simulink model "ResolvedMotion_Example"  (R2015b)
settings: Solver=ode45  StartTime=0.0  StopTime=10.0  MaxStep=1e-2  RelTol=1e-9  AbsTol=1e-9
InitFcn:
  | ResolvedMotion_Example_Init
values from neighbouring files (symbols this model uses):
  M0 = H0*q0dot0+H0m*qmdot0    [ResolvedMotion_Example_Init.m]
  qmdot0 = zeros(4,1)    [ResolvedMotion_Example_Init.m]
libraries: SPART_Lib x3, aerolibtransform2 x2, simulink x1
settings Model: Creator=Josep  LastModifiedBy=Josep
settings DataIOCC: SaveFormat=Array
settings HardwareCC: ProdBitPerPointer=32  ProdLargestAtomicFloat=None  ProdIntDivRoundTo=Undefined  ProdEndianess=Unspecified  ProdWordSize=32  ProdHWDeviceType=32-bit Generic
settings GRTTargetCC: GeneratePreprocessorConditionals=Disable all
settings ConfigComp: CovModelRefEnable=Off

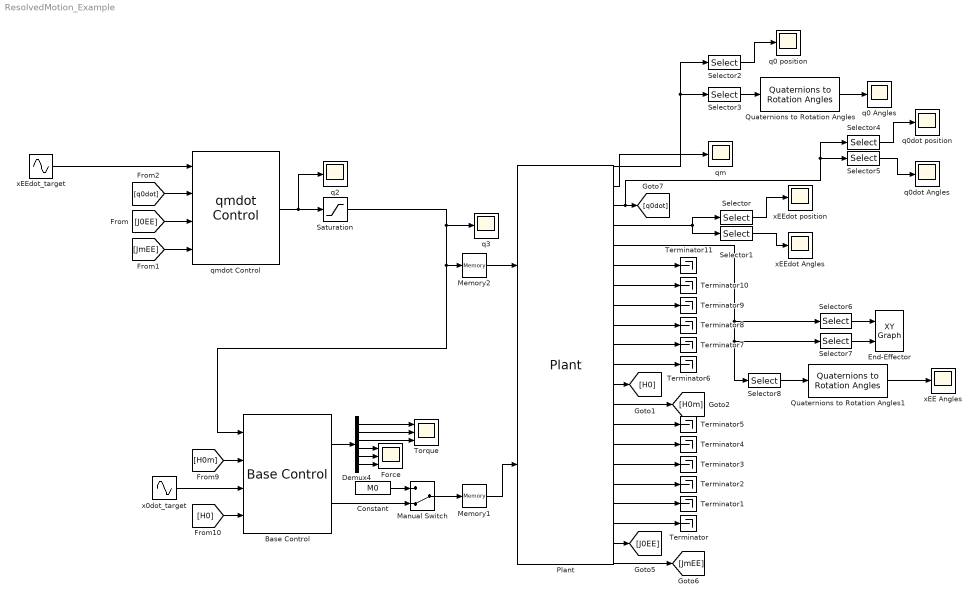
== system ResolvedMotion_Example ==
  Base Control : SPART_Lib/Control/Base Control
  Constant : Constant  Value=M0
  Demux4 : Demux  Outputs=6
  End-Effector : simulink/Sinks/XY Graph  xmin=3.5  xmax=4  ymin=-0.25  ymax=0.25  st=-1
  Force : Scope  NumInputPorts=3
  Manual Switch : ManualSwitch  CurrentSetting=0
  Memory1 : Memory  X0=M0  InheritSampleTime=on
  Memory2 : Memory  X0=qmdot0  InheritSampleTime=on
  Plant : SPART_Lib/Plant
  Quaternions to Rotation Angles : aerolibtransform2/Quaternions to Rotation Angles  rotationOrder=XYZ
  Quaternions to Rotation Angles1 : aerolibtransform2/Quaternions to Rotation Angles  rotationOrder=XYZ
  Saturation : Saturate  UpperLimit=1  LowerLimit=-1
  Selector : Selector  InputPortWidth=6  IndexOptions=Index vector (dialog)  Indices=[4:6]  OutputSizes=1
  Selector1 : Selector  InputPortWidth=6  IndexOptions=Index vector (dialog)  Indices=[1:3]  OutputSizes=1
  Selector2 : Selector  InputPortWidth=7  IndexOptions=Index vector (dialog)  Indices=[5:7]  OutputSizes=1
  Selector3 : Selector  InputPortWidth=7  IndexOptions=Index vector (dialog)  Indices=[4,1:3]  OutputSizes=1
  Selector4 : Selector  InputPortWidth=6  IndexOptions=Index vector (dialog)  Indices=[4:6]  OutputSizes=1
  Selector5 : Selector  InputPortWidth=6  IndexOptions=Index vector (dialog)  Indices=[1:3]  OutputSizes=1
  Selector6 : Selector  InputPortWidth=7  IndexOptions=Index vector (dialog)  Indices=[5]  OutputSizes=1
  Selector7 : Selector  InputPortWidth=7  IndexOptions=Index vector (dialog)  Indices=[6]  OutputSizes=1
  Selector8 : Selector  InputPortWidth=7  IndexOptions=Index vector (dialog)  Indices=[4,1:3]  OutputSizes=1
  Terminator{,1..11} (12 alike) : Terminator
  Torque : Scope  NumInputPorts=3
  q0 Angles : Scope
  "q0 position " : Scope
  q0dot Angles : Scope
  q0dot position : Scope
  q2 : Scope
  q3 : Scope
  qm : Scope
  qmdot Control : SPART_Lib/Control/qmdot Control
  x0dot_target : Sin  Amplitude=[0;0;0.1;0;0;0]  Frequency=pi/4  SampleTime=0
  xEE Angles : Scope
  xEEdot Angles : Scope
  xEEdot position : Scope
  xEEdot_target : Sin  Amplitude=[0;0;0.1;0.05;0.05;0]  Frequency=pi/2  Phase=[0;0;0;0;pi/2;0]  SampleTime=0
  wires:
  Plant/12 -> [H0]
  Plant/20 -> [J0EE]
  Plant/21 -> [JmEE]
  [H0m] -> Base Control/2
  x0dot_target/1 -> Base Control/3
  [H0] -> Base Control/4
  Constant/1 -> Manual Switch/1
  Demux4/1 -> Torque/1
  Demux4/2 -> Torque/2
  Demux4/3 -> Torque/3
  Demux4/4 -> Force/1
  Demux4/5 -> Force/2
  Demux4/6 -> Force/3
  xEEdot_target/1 -> qmdot Control/1
  [J0EE] -> qmdot Control/3
  [JmEE] -> qmdot Control/4
  qmdot Control/1 -> q2/1, Saturation/1
  Base Control/2 -> Manual Switch/2
  Memory1/1 -> Plant/2
  Manual Switch/1 -> Memory1/1
  Base Control/1 -> Demux4/1
  [q0dot] -> qmdot Control/2
  Plant/19 -> Terminator/1
  Plant/18 -> Terminator1/1
  Plant/17 -> Terminator2/1
  Plant/16 -> Terminator3/1
  Plant/15 -> Terminator4/1
  Plant/13 -> [H0m]
  Plant/14 -> Terminator5/1
  Plant/11 -> Terminator6/1
  Plant/10 -> Terminator7/1
  Plant/9 -> Terminator8/1
  Plant/8 -> Terminator9/1
  Plant/7 -> Terminator10/1
  Plant/6 -> Terminator11/1
  Plant/5 -> Selector6/1, Selector7/1, Selector8/1
  Plant/4 -> Selector1/1, Selector/1
  Selector/1 -> xEEdot position/1
  Plant/1 -> Selector2/1, Selector3/1
  Selector2/1 -> "q0 position "/1
  Selector3/1 -> Quaternions to Rotation Angles/1
  Plant/3 -> Selector4/1, Selector5/1, [q0dot]
  Selector4/1 -> q0dot position/1
  Selector5/1 -> q0dot Angles/1
  Plant/2 -> qm/1
  Saturation/1 -> Memory2/1, Base Control/1, q3/1
  Memory2/1 -> Plant/1
  Selector6/1 -> End-Effector/1
  Selector7/1 -> End-Effector/2
  Quaternions to Rotation Angles/1 -> q0 Angles/1
  Selector1/1 -> xEEdot Angles/1
  Selector8/1 -> Quaternions to Rotation Angles1/1
  Quaternions to Rotation Angles1/1 -> xEE Angles/1
